simulink model "Furuta_Control_all_states"  (R2018a)
settings: Solver=FixedStepAuto  StartTime=0.0  StopTime=50  FixedStep=Ts  RelTol=1e-3
PreLoadFcn:
  | %myBusDef
StartFcn:
  | % Full path to the block
  | %blk = 'Furuta_Control/Bus Creator';
  | 
  | % Attach the event listener
  | %h = add_exec_event_listener(blk, ...
  | %         'PostOutputs', @displayBusdata);
values from neighbouring files (symbols this model uses):
  alpha = J + (M+m1/3+m2)*L1^2    (= 0.001331208)    [CoSim_Furuta.m]    (also in Furuta_Constants.m)
  beta = (M + m2/3)*L2^2    (= 0.001321592)    [CoSim_Furuta.m]    (also in Furuta_Constants.m)
  gamma = (M + m2/2)*L2*L1    (= 0.000684156)    [CoSim_Furuta.m]    (also in Furuta_Constants.m)
  GSwingUp = 3    [CoSim_Furuta.m]    (also in Furuta_Constants.m = 2.4738)
  initial_state = pi    (= 3.14159265359)    [CoSim_Furuta.m]    (also in Furuta_Constants.m)
  K = x    [CoSim_Furuta.m]
  kb_m = 6.75e-4    (= 0.000675)    [CoSim_Furuta.m]    (also in Furuta_Constants.m)
  kb_p = 4.7940e-04    (= 0.0004794)    [CoSim_Furuta.m]    (also in Furuta_Constants.m)
  ke = 0.5    [CoSim_Furuta.m]    (also in Furuta_Constants.m)
  Re = 14.5    [CoSim_Furuta.m]    (also in Furuta_Constants.m)
  sigma = (M + m2/2)*g*L2    (= 0.10169046)    [CoSim_Furuta.m]    (also in Furuta_Constants.m)
settings Model: Creator=Marcelo  LastModifiedBy=Felipe
settings SolverCC: ZeroCrossControl=DisableAll
settings DebuggingCC: ParameterOverflowMsg=warning  BusObjectLabelMismatch=error
settings ModelReferenceCC: ModelReferenceMinAlgLoopOccurrences=on
settings CodeAppCC: StateflowObjectComments=on
settings ConfigComp: PLC_TargetIDE=codesys23  PLC_GenerateReport=off  PLC_LaunchReport=off

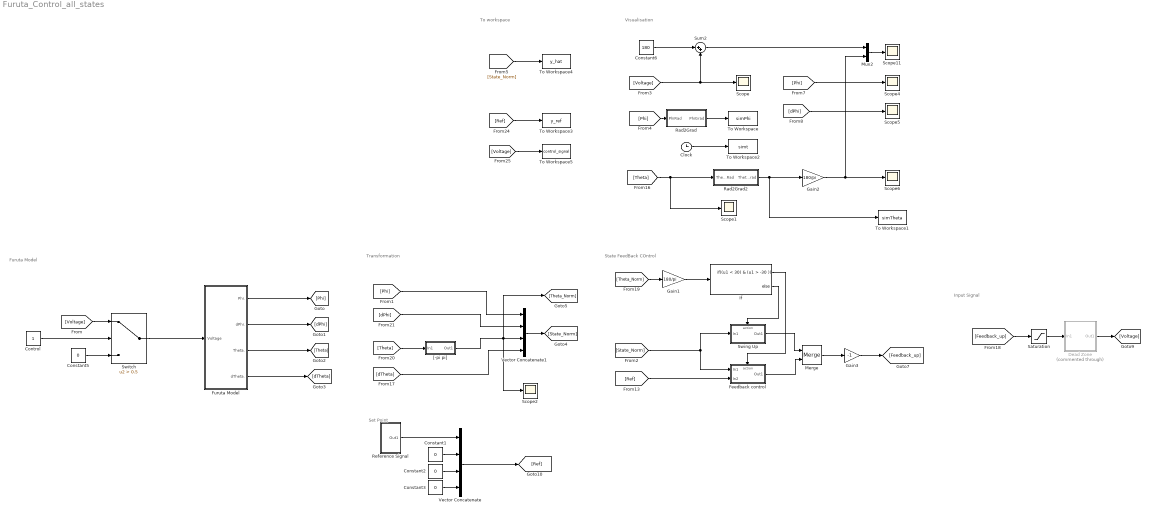
== system Furuta_Control_all_states ==
  note: To workspace
  note: Transformation
  note: State FeedBack COntrol
  note: Input Signal
  note: Furuta Model
  note: Visualisation
  note: Set Point
  Clock : Clock
  Constant{1..3,5} (4 alike) : Constant  Value=0
  Constant6 : Constant  Value=180
  Control : Constant
  Dead Zone : Subsystem  Commented=through
  Feedback control : Subsystem  TreatAsAtomicUnit=on
  "Furuta Model " : Subsystem
  Gain1 : Gain  Gain=180/pi
  Gain2 : Gain  Gain=180/pi
  Gain3 : Gain  Gain=-1
  If : If  IfExpression=(u1 < 30) & (u1 > -30 )
  Merge : Merge
  Mux2 : Mux  Inputs=2
  Rad2Grad : Subsystem
  Rad2Grad2 : Subsystem
  Reference Signal : Subsystem
  Saturation : Saturate  UpperLimit=6  LowerLimit=-6
  Scope{,1..2,4..6,11} (7 alike) : Scope
  Sum2 : Sum  Inputs=|++
  Swing Up : Subsystem  TreatAsAtomicUnit=on
  Switch : Switch  Criteria=u2 > Threshold  Threshold=0.5
  To Workspace : ToWorkspace  VariableName=simPhi  SampleTime=-1
      settings: Save2DSignal=2-D array (concatenate along first dimension)
  To Workspace1 : ToWorkspace  VariableName=simTheta  SampleTime=-1
      settings: Save2DSignal=2-D array (concatenate along first dimension)
  To Workspace2 : ToWorkspace  VariableName=simt  SampleTime=-1
      settings: Save2DSignal=2-D array (concatenate along first dimension)
  To Workspace3 : ToWorkspace  VariableName=y_ref  SampleTime=-1
      settings: Save2DSignal=2-D array (concatenate along first dimension)
  To Workspace4 : ToWorkspace  VariableName=y_hat  SampleTime=-1
      settings: Save2DSignal=2-D array (concatenate along first dimension)
  To Workspace5 : ToWorkspace  VariableName=control_signal  SampleTime=-1
      settings: Save2DSignal=2-D array (concatenate along first dimension)
  Vector Concatenate : Concatenate  NumInputs=4
  Vector Concatenate1 : Concatenate  NumInputs=4
  "[-pi pi]" : Subsystem
  wires:
  "Furuta Model "/1(Phi.) -> [Phi]
  "Furuta Model "/2(dPhi.) -> [dPhi]
  [Voltage] -> Sum2/2, Scope/1
  [Phi] -> Scope4/1
  [dPhi] -> Scope5/1
  [Theta] -> "[-pi pi]"/1(In1)
  Rad2Grad2/1(ThetaGrad) -> To Workspace1/1, Gain2/1
  Clock/1 -> To Workspace2/1
  Rad2Grad/1(PhiGrad) -> To Workspace/1
  If/2 -> Swing Up/Action
  Swing Up/1(Out1) -> Merge/1
  If/1 -> Feedback control/Action
  Gain2/1 -> Scope6/1, Mux2/2
  "Furuta Model "/4(dTheta.) -> [dTheta]
  [dTheta] -> Vector Concatenate1/4
  Feedback control/1(Out1) -> Merge/2
  [Voltage] -> Switch/1
  Control/1 -> Switch/2
  Constant5/1 -> Switch/3
  [Phi] -> Rad2Grad/1(PhiRad)
  Constant6/1 -> Sum2/1
  Mux2/1 -> Scope11/1
  Sum2/1 -> Mux2/1
  "Furuta Model "/3(Theta.) -> [Theta]
  [dPhi] -> Vector Concatenate1/2
  [Phi] -> Vector Concatenate1/1
  Vector Concatenate1/1 -> [State_Norm]
  "[-pi pi]"/1(Out1) -> Scope2/1, [Theta_Norm], Vector Concatenate1/3
  [State_Norm] -> Feedback control/1(In1), Swing Up/1(In1)
  [Theta_Norm] -> Gain1/1
  Gain1/1 -> If/1
  Dead Zone/1(Out1) -> [Voltage]
  [Feedback_up] -> Saturation/1
  Saturation/1 -> Dead Zone/1(In1)
  Merge/1 -> Gain3/1
  Gain3/1 -> [Feedback_up]
  [Theta] -> Scope1/1, Rad2Grad2/1(ThetaRad)
  Switch/1 -> "Furuta Model "/1("Voltage ")
  Reference Signal/1(Out1) -> Vector Concatenate/1
  Vector Concatenate/1 -> [Ref]
  Constant1/1 -> Vector Concatenate/2
  Constant2/1 -> Vector Concatenate/3
  Constant3/1 -> Vector Concatenate/4
  [Ref] -> Feedback control/2(In2)
  [Ref] -> To Workspace3/1
  [Voltage] -> To Workspace5/1
  [State_Norm] -> To Workspace4/1

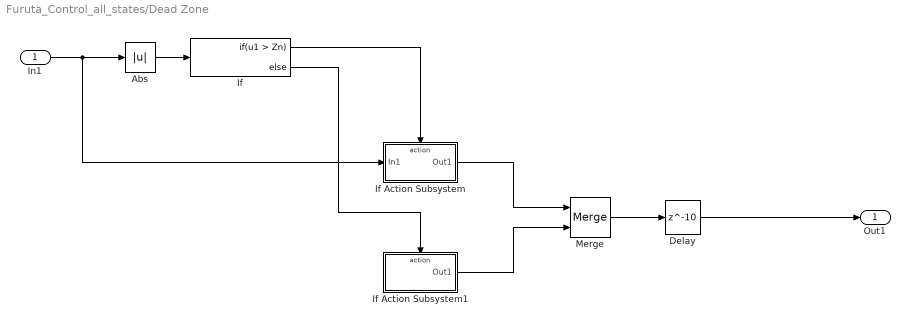
== system Furuta_Control_all_states/Dead Zone ==
  In1 : Inport
  Abs : Abs
  Delay : Delay  DelayLength=10
  If : If  IfExpression=u1 > Zn
  If Action Subsystem : Subsystem  TreatAsAtomicUnit=on
  If Action Subsystem1 : Subsystem  TreatAsAtomicUnit=on
  Merge : Merge
  Out1 : Outport
  wires:
  Delay/1 -> Out1/1
  Merge/1 -> Delay/1
  If Action Subsystem1/1(Out1) -> Merge/2
  If Action Subsystem/1(Out1) -> Merge/1
  If/2 -> If Action Subsystem1/Action
  If/1 -> If Action Subsystem/Action
  Abs/1 -> If/1
  In1/1 -> Abs/1, If Action Subsystem/1(In1)

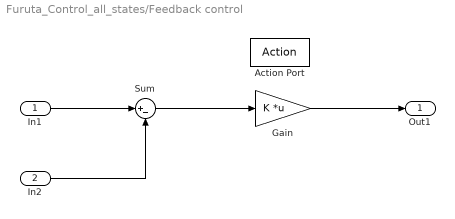
== system Furuta_Control_all_states/Feedback control ==
  In1 : Inport
  In2 : Inport  Port=2
  Action Port : ActionPort  ActionType=then
  Gain : Gain  Gain=K  Multiplication=Matrix(K*u)  ParamDataTypeStr=double  OutDataTypeStr=double
  Sum : Sum  Inputs=|+-
  Out1 : Outport
  wires:
  Gain/1 -> Out1/1
  Sum/1 -> Gain/1
  In1/1 -> Sum/1
  In2/1 -> Sum/2

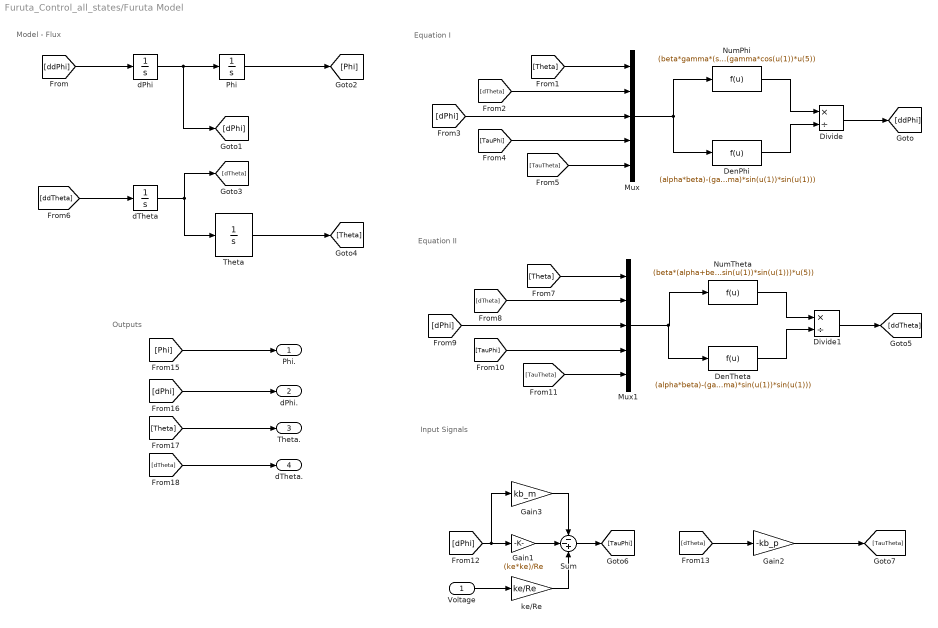
== system Furuta_Control_all_states/Furuta Model  ==
  note: Outputs
  note: Input Signals
  note: Equation II
  note: Equation I
  note: Model - Flux
  "Voltage " : Inport
  DenPhi : Fcn  Expr=(alpha*beta)-(gamma*gamma)+((beta*beta+gamma*gamma)*sin(u(1))*sin(u(1)))
  DenTheta : Fcn  Expr=(alpha*beta)-(gamma*gamma)+((beta*beta+gamma*gamma)*sin(u(1))*sin(u(1)))
  Divide : Product  Inputs=*/
  Divide1 : Product  Inputs=*/
  Gain1 : Gain  Gain=(ke*ke)/Re
  Gain2 : Gain  Gain=-kb_p
  Gain3 : Gain  Gain=kb_m
  Mux : Mux  Inputs=5
  Mux1 : Mux  Inputs=5
  NumPhi : Fcn  Expr=(beta*gamma*(sin(u(1))*sin(u(1))-1)*sin(u(1))*u(3)*u(3))-(2*beta*beta*cos(u(1))*sin(u(1))*u(3)*u(2))+(beta*gamma*sin(u(1))*u(2)*u(2))-(gamma*sigma*cos(u(1))*sin(u(1)))+(beta*u(4))-(gamma*cos(u(1))*u(5))
  NumTheta : Fcn  Expr=(beta*(alpha+beta*sin(u(1))*sin(u(1)))*cos(u(1))*sin(u(1))*u(3)*u(3))+(2*beta*gamma*(1-sin(u(1))*sin(u(1)))*sin(u(1))*u(3)*u(2))-(gamma*gamma*cos(u(1))*sin(u(1))*u(2)*u(2))+(sigma*(alpha+beta*sin(u(1))*sin(u(1)))*sin(u(1)))-(gamma*cos(u(1))*u(4))+((alpha+beta*sin(u(1))*sin(u(1)))*u(5))
  Phi : Integrator
  Sum : Sum  Inputs=--+
  Theta : Integrator  InitialCondition=initial_state
  dPhi : Integrator
  dTheta : Integrator
  "ke/Re " : Gain  Gain=ke/Re
  Phi. : Outport
  dPhi. : Outport  Port=2
  Theta. : Outport  Port=3
  dTheta. : Outport  Port=4
  wires:
  Divide/1 -> [ddPhi]
  "ke/Re "/1 -> Sum/3
  Sum/1 -> [TauPhi]
  Gain1/1 -> Sum/2
  "Voltage "/1 -> "ke/Re "/1
  [dTheta] -> Gain2/1
  Gain3/1 -> Sum/1
  dTheta/1 -> [dTheta], Theta/1
  Theta/1 -> [Theta]
  [Theta] -> Mux1/1
  Mux1/1 -> DenTheta/1, NumTheta/1
  [dTheta] -> Mux1/2
  [dPhi] -> Mux1/3
  [TauTheta] -> Mux1/5
  [TauPhi] -> Mux1/4
  [Theta] -> Mux/1
  [TauTheta] -> Mux/5
  [TauPhi] -> Mux/4
  Phi/1 -> [Phi]
  [dPhi] -> Mux/3
  DenPhi/1 -> Divide/2
  [ddPhi] -> dPhi/1
  [ddTheta] -> dTheta/1
  dPhi/1 -> [dPhi], Phi/1
  NumTheta/1 -> Divide1/1
  NumPhi/1 -> Divide/1
  DenTheta/1 -> Divide1/2
  Mux/1 -> DenPhi/1, NumPhi/1
  [dPhi] -> Gain3/1, Gain1/1
  [dTheta] -> Mux/2
  Divide1/1 -> [ddTheta]
  [Phi] -> Phi./1
  [dPhi] -> dPhi./1
  [Theta] -> Theta./1
  [dTheta] -> dTheta./1
  Gain2/1 -> [TauTheta]

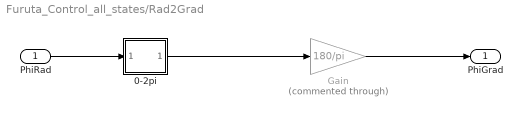
== system Furuta_Control_all_states/Rad2Grad ==
  PhiRad : Inport
  0-2pi : Subsystem
  Gain : Gain  Commented=through  Gain=180/pi
  PhiGrad : Outport
  wires:
  0-2pi/1(Out1) -> Gain/1
  Gain/1 -> PhiGrad/1
  PhiRad/1 -> 0-2pi/1(In1)

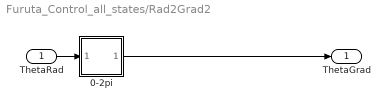
== system Furuta_Control_all_states/Rad2Grad2 ==
  ThetaRad : Inport
  0-2pi : Subsystem
  ThetaGrad : Outport
  wires:
  ThetaRad/1 -> 0-2pi/1(In1)
  0-2pi/1(Out1) -> ThetaGrad/1

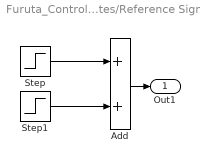
== system Furuta_Control_all_states/Reference Signal ==
  Add : Sum
  Step : Step  Time=15  After=pi/2  SampleTime=0
  Step1 : Step  Time=35  After=-pi  SampleTime=0
  Out1 : Outport
  wires:
  Step/1 -> Add/1
  Add/1 -> Out1/1
  Step1/1 -> Add/2

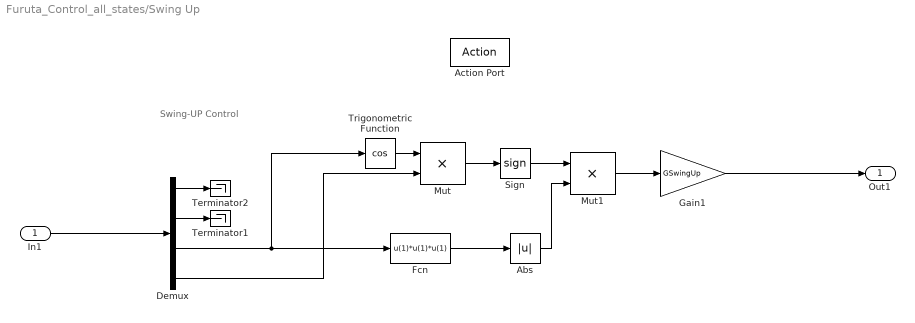
== system Furuta_Control_all_states/Swing Up ==
  note: Swing-UP Control
  In1 : Inport
  Action Port : ActionPort  ActionType=else
  Abs : Abs
  Demux : Demux
  Fcn : Fcn  Expr=u(1)*u(1)*u(1)
  Gain1 : Gain  Gain=GSwingUp
  Mut : Product  Inputs=**
  Mut1 : Product  Inputs=**
  Sign : Signum
  Terminator1 : Terminator
  Terminator2 : Terminator
  Trigonometric Function : Trigonometry  Operator=cos
  Out1 : Outport  InitialOutput=0
  wires:
  Gain1/1 -> Out1/1
  Demux/2 -> Terminator1/1
  Demux/1 -> Terminator2/1
  Mut1/1 -> Gain1/1
  Fcn/1 -> Abs/1
  Trigonometric Function/1 -> Mut/1
  Demux/4 -> Mut/2
  Abs/1 -> Mut1/2
  Sign/1 -> Mut1/1
  Mut/1 -> Sign/1
  Demux/3 -> Fcn/1, Trigonometric Function/1
  In1/1 -> Demux/1

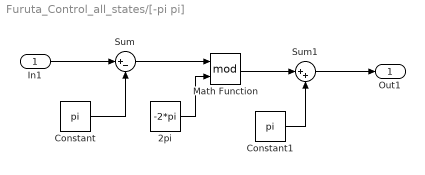
== system Furuta_Control_all_states/[-pi pi] ==
  In1 : Inport
  2pi : Constant  Value=-2*pi
  Constant : Constant  Value=pi
  Constant1 : Constant  Value=pi
  Math Function : Math  Operator=mod  SaturateOnIntegerOverflow=on
  Sum : Sum  Inputs=|+-
  Sum1 : Sum  Inputs=|++
  Out1 : Outport
  wires:
  2pi/1 -> Math Function/2
  In1/1 -> Sum/1
  Sum/1 -> Math Function/1
  Constant/1 -> Sum/2
  Constant1/1 -> Sum1/2
  Sum1/1 -> Out1/1
  Math Function/1 -> Sum1/1

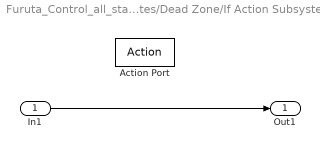
== system Furuta_Control_all_states/Dead Zone/If Action Subsystem ==
  In1 : Inport
  Action Port : ActionPort  ActionType=then
  Out1 : Outport
  wires:
  In1/1 -> Out1/1

== system Furuta_Control_all_states/Dead Zone/If Action Subsystem1 ==
  Action Port : ActionPort  ActionType=else
  Constant : Constant  Value=0
  Out1 : Outport
  wires:
  Constant/1 -> Out1/1

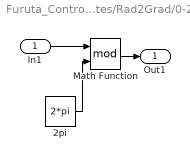
== system Furuta_Control_all_states/Rad2Grad/0-2pi ==
  In1 : Inport
  2pi : Constant  Value=2*pi
  Math Function : Math  Operator=mod  SaturateOnIntegerOverflow=on
  Out1 : Outport
  wires:
  2pi/1 -> Math Function/2
  Math Function/1 -> Out1/1
  In1/1 -> Math Function/1

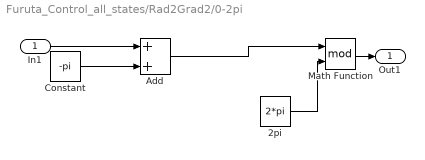
== system Furuta_Control_all_states/Rad2Grad2/0-2pi ==
  In1 : Inport
  2pi : Constant  Value=2*pi
  Add : Sum
  Constant : Constant  Value=-pi
  Math Function : Math  Operator=mod  SaturateOnIntegerOverflow=on
  Out1 : Outport
  wires:
  Math Function/1 -> Out1/1
  2pi/1 -> Math Function/2
  Constant/1 -> Add/2
  In1/1 -> Add/1
  Add/1 -> Math Function/1
